simulink model "mloc_estimation_postprocessing"  (R2018b)
settings: configuration reference "Active" (kept outside this file)
model workspace (MAT data in the model file):
  P_VDC_LocalizationMode = Simulink.Parameter
  P_VDC_LocalizationMode.Value = 1
  P_VDC_LocalizationMode.DataType = 'auto'
  P_VDC_LocalizationMode.Dimensions = [1 1]
undefined symbols (not defined in the file): l_front_m, l_rear_m, P_MLOC_MaxWheelslip_perc, P_MLOC_MaxWheelslipangle_rad, P_MLOC_MinWheelslip_perc, P_MLOC_MinWheelslipangle_rad, P_MLOC_OdometryMode, P_MLOC_OdometrySwitchSpeed_mps, P_MLOC_VLOCManualReset_psi_rad, P_MLOC_VLOCManualReset_x_m, P_MLOC_VLOCManualReset_y_m, P_MLOC_VLOCResetMode, P_VDC_CurvatureEstimateMax_radpm, P_VDC_CurvatureEstimationMode, P_VDC_LowPassT1Curvature, P_VDC_MinVelSlipCalc_mps, P_VDC_resLim_dGPS_m, P_VDC_resLim_dVLOC_m, P_VDC_resLim_psiGPS_rad, P_VDC_resLim_psiVLOC_rad, P_VDC_resLim_sGPS_m, P_VDC_resLim_sVLOC_m, P_VDC_resLim_vx_mps, P_VDC_resLim_vy_mps, tS, TUMOdometryEstimationState, TUMStateEstimationState, tw_front_m, tw_rear_m, tyreradius_front_m, tyreradius_rear_m
libraries: simulink x11, rr_general x4
settings Model: DataDictionary=mloc_estimation_postprocessing.sldd  ParameterArgumentNames=P_VDC_LocalizationMode  Creator=wischnewski  LastModifiedBy=ge34qer

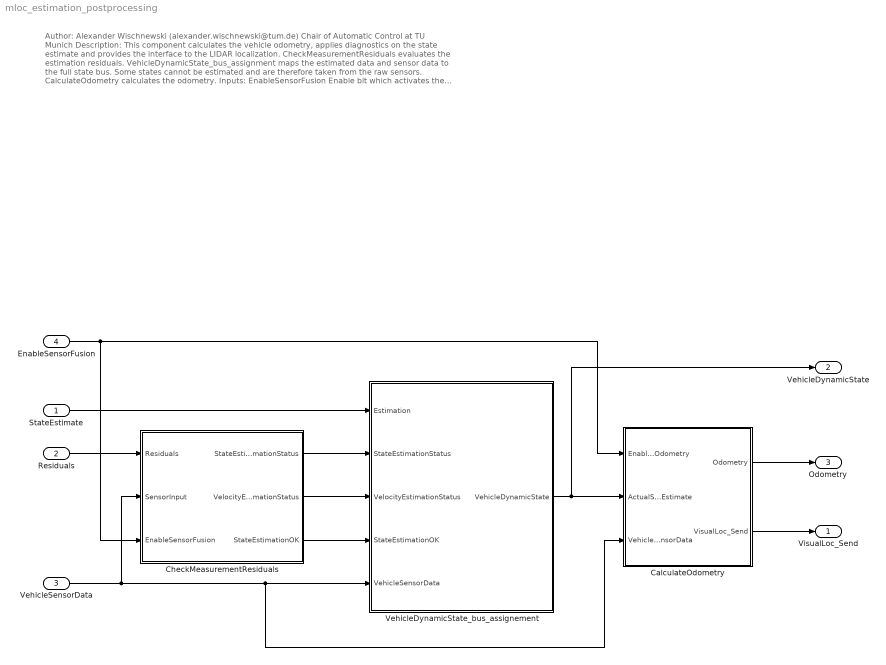
== system mloc_estimation_postprocessing ==
  note: Author: Alexander Wischnewski (alexander.wischnewski@tum.de)
      | Chair of Automatic Control at TU Munich
      |
      | Description: This component calculates the vehicle odometry, applies diagnostics on the state estimate and provides the interface to the LIDAR localization.
      |
      | CheckMeasurementResiduals evaluates the estimation residuals.
      |
      | VehicleDynamicState_bus_assignment maps the estimated data and sensor data to the full state bus. Some states cannot be estimated and are therefore taken from the raw sensors.
      |
      | CalculateOdometry calculates the odometry.
      |
      | Inputs:
      | EnableSensorFusion Enable bit which activates the Kalman Filter
      | StateEstimate State estimation vector from the Kalman Filter
      | Residuals Residual vector of the Kalman Filter
      | VehicleSensorData raw sensor data
      |
      | Outputs:
      | VehicleDynamicState Estimate of the vehicle dynamic state (best available)
      | VisualLocSend Data which is send to the LIDAR localization algorithm
      | Odometry Vehicle odometry as forward integrated position
  "StateEstimate " : Inport  OutDataTypeStr=Bus: StateEstimation_state  BusOutputAsStruct=on
  Residuals : Inport  Port=2  OutDataTypeStr=Bus: StateEstimation_residuals  BusOutputAsStruct=on
  VehicleSensorData : Inport  Port=3  OutDataTypeStr=Bus: VehicleSensorData  BusOutputAsStruct=on
  EnableSensorFusion : Inport  Port=4  OutDataTypeStr=boolean  BusOutputAsStruct=on
  CalculateOdometry : Subsystem
  CheckMeasurementResiduals : Subsystem
  VehicleDynamicState_bus_assignement : Subsystem
  VisualLoc_Send : Outport  OutDataTypeStr=Bus: VisualLoc_Send  BusOutputAsStruct=on
  VehicleDynamicState : Outport  Port=2  OutDataTypeStr=Bus: VehicleDynamicState  BusOutputAsStruct=on
  Odometry : Outport  Port=3  OutDataTypeStr=Bus: Odometry  BusOutputAsStruct=on
  wires:
  VehicleDynamicState_bus_assignement/1(VehicleDynamicState) -> VehicleDynamicState/1, CalculateOdometry/2(ActualStateEstimate)
  CalculateOdometry/2(VisualLoc_Send) -> VisualLoc_Send/1
  EnableSensorFusion/1 -> CalculateOdometry/1(EnableOdometry), CheckMeasurementResiduals/3(EnableSensorFusion)
  CheckMeasurementResiduals/1(StateEstimationStatus) -> VehicleDynamicState_bus_assignement/2(StateEstimationStatus)
  CheckMeasurementResiduals/2(VelocityEstimationStatus) -> VehicleDynamicState_bus_assignement/3(VelocityEstimationStatus)
  CheckMeasurementResiduals/3(StateEstimationOK) -> VehicleDynamicState_bus_assignement/4(StateEstimationOK)
  "StateEstimate "/1 -> VehicleDynamicState_bus_assignement/1(Estimation)
  CalculateOdometry/1(Odometry) -> Odometry/1
  VehicleSensorData/1 -> CheckMeasurementResiduals/2(SensorInput), CalculateOdometry/3(VehicleSensorData), VehicleDynamicState_bus_assignement/5(VehicleSensorData)
  Residuals/1 -> CheckMeasurementResiduals/1(Residuals)

== system mloc_estimation_postprocessing/CalculateOdometry ==
  note: calculates an Odometry based on
      | the vehicle motion sensors. Different options are available.
      | Check "Integrate Odometry" for details.
  EnableOdometry : Inport
  ActualStateEstimate : Inport  Port=2
  VehicleSensorData : Inport  Port=3
  DetermineResetPosition : Subsystem
  IntegrateOdometry : Subsystem
  VisualLocalizationInterface : Subsystem
  Odometry : Outport
  VisualLoc_Send : Outport  Port=2  OutDataTypeStr=Bus: VisualLoc_Send  BusOutputAsStruct=on
  wires:
  IntegrateOdometry/1(Odometry) -> VisualLocalizationInterface/1(Odometry), Odometry/1
  DetermineResetPosition/2(ResetPositionValid_b) -> VisualLocalizationInterface/3(ResetPosition_Valid), IntegrateOdometry/4(ResetPositionValid)
  DetermineResetPosition/1(ResetPosition) -> VisualLocalizationInterface/2(ResetPosition), IntegrateOdometry/3(ResetPosition)
  VehicleSensorData/1 -> VisualLocalizationInterface/5(VehicleSensorData), IntegrateOdometry/5(VehicleSensors), DetermineResetPosition/2(VehicleSensorData)
  EnableOdometry/1 -> IntegrateOdometry/1(EnableOdometry)
  ActualStateEstimate/1 -> VisualLocalizationInterface/4(VehicleDynamicState), IntegrateOdometry/2(ActualStateEstimate), DetermineResetPosition/1(StateEstimate)
  VisualLocalizationInterface/1(VisualLoc_Send) -> VisualLoc_Send/1

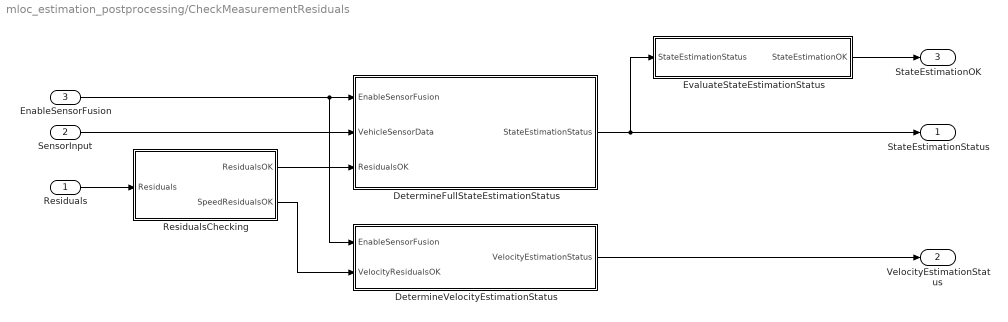
== system mloc_estimation_postprocessing/CheckMeasurementResiduals ==
  Residuals : Inport
  SensorInput : Inport  Port=2
  EnableSensorFusion : Inport  Port=3
  DetermineFullStateEstimationStatus : Subsystem
  DetermineVelocityEstimationStatus : Subsystem
  EvaluateStateEstimationStatus : Subsystem
  ResidualsChecking : Subsystem
  StateEstimationStatus : Outport
  VelocityEstimationStatus : Outport  Port=2
  StateEstimationOK : Outport  Port=3
  wires:
  Residuals/1 -> ResidualsChecking/1(Residuals)
  EnableSensorFusion/1 -> DetermineVelocityEstimationStatus/1(EnableSensorFusion), DetermineFullStateEstimationStatus/1(EnableSensorFusion)
  EvaluateStateEstimationStatus/1(StateEstimationOK) -> StateEstimationOK/1
  ResidualsChecking/2(SpeedResidualsOK) -> DetermineVelocityEstimationStatus/2(VelocityResidualsOK)
  DetermineVelocityEstimationStatus/1(VelocityEstimationStatus) -> VelocityEstimationStatus/1
  DetermineFullStateEstimationStatus/1(StateEstimationStatus) -> StateEstimationStatus/1, EvaluateStateEstimationStatus/1(StateEstimationStatus)
  SensorInput/1 -> DetermineFullStateEstimationStatus/2(VehicleSensorData)
  ResidualsChecking/1(ResidualsOK) -> DetermineFullStateEstimationStatus/3(ResidualsOK)

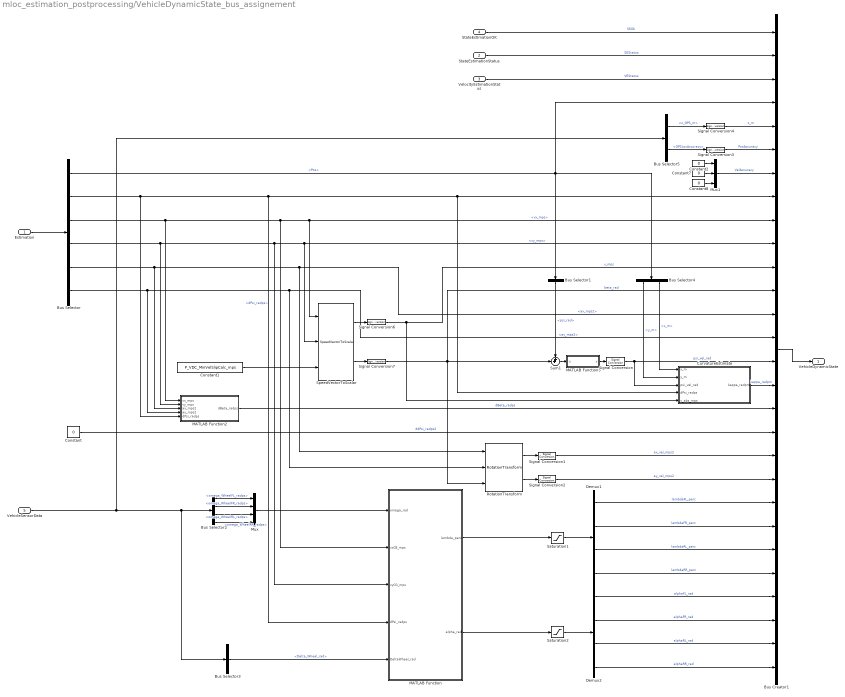
== system mloc_estimation_postprocessing/VehicleDynamicState_bus_assignement ==
  Estimation : Inport
  StateEstimationStatus : Inport  Port=2
  VelocityEstimationStatus : Inport  Port=3
  StateEstimationOK : Inport  Port=4
  VehicleSensorData : Inport  Port=5
  Bus Creator1 : BusCreator  Inputs=28
  Bus Selector : BusSelector  OutputSignals=Pos,dPsi_radps,vx_mps,vy_mps,ax_mps2,ay_mps2
  Bus Selector1 : BusSelector  OutputSignals=psi_rad
  Bus Selector2 : BusSelector  OutputSignals=omega_WheelFL_radps,omega_WheelFR_radps,omega_WheelRL_radps,omega_WheelRR_radps
  Bus Selector3 : BusSelector  OutputSignals=Delta_Wheel_rad
  Bus Selector4 : BusSelector  OutputSignals=y_m,x_m
  Bus Selector5 : BusSelector  OutputSignals=z_GPS_m,GPSLocAccuracy
  Constant{,2,7..8} (4 alike) : Constant  Value=0
  Constant1 : Constant  Value=P_VDC_MinVelSlipCalc_mps
  CurvatureEstimate : Subsystem
  Demux1 : Demux
  Demux2 : Demux
  MATLAB Function : MATLAB Function  TreatAsAtomicUnit=on
  MATLAB Function2 : MATLAB Function  TreatAsAtomicUnit=on
  MATLAB Function3 : MATLAB Function  TreatAsAtomicUnit=on
  Mux : Mux
  Mux1 : Mux  Inputs=3
  RotationTransform : rr_general/RotationTransform  SystemSampleTime=-1
  Saturation1 : Saturate  UpperLimit=P_MLOC_MaxWheelslip_perc  LowerLimit=P_MLOC_MinWheelslip_perc
  Saturation2 : Saturate  UpperLimit=P_MLOC_MaxWheelslipangle_rad  LowerLimit=P_MLOC_MinWheelslipangle_rad
  Signal Conversion{,1..4,6..7} (7 alike) : SignalConversion  OverrideOpt=off
  SpeedVectorToScalar : rr_general/SpeedVectorToScalar  SystemSampleTime=-1
  Sum1 : Sum  Inputs=++|
  VehicleDynamicState : Outport
  wires:
  Bus Creator1/1 -> VehicleDynamicState/1
  Sum1/1 -> MATLAB Function3/1(u)
  Bus Selector/3 -> MATLAB Function2/1(vx_mps), MATLAB Function/2(vxCB_mps), SpeedVectorToScalar/1, Bus Creator1/9  "<vx_mps>"
  Bus Selector/1 -> Bus Selector4/1, Bus Creator1/4, Bus Selector1/1  "<Pos>"
  Bus Selector1/1 -> Sum1/1  "<psi_rad>"
  Estimation/1 -> Bus Selector/1
  StateEstimationStatus/1 -> Bus Creator1/2  "SEStatus"
  MATLAB Function3/1(y) -> Signal Conversion/1
  CurvatureEstimate/1(kappa_radpm) -> Bus Creator1/16  "kappa_radpm"
  Signal Conversion/1 -> Bus Creator1/15, CurvatureEstimate/3(psi_vel_rad)  "psi_vel_rad"
  MATLAB Function2/1(dBeta_radps) -> Bus Creator1/17  "dBeta_radps"
  Constant/1 -> Bus Creator1/18  "ddPsi_radps2"
  Bus Selector/4 -> MATLAB Function/3(vyCG_mps), Bus Creator1/10, SpeedVectorToScalar/2, MATLAB Function2/2(vy_mps)  "<vy_mps>"
  SpeedVectorToScalar/1 -> Signal Conversion6/1
  SpeedVectorToScalar/2 -> Signal Conversion7/1
  Signal Conversion6/1 -> Bus Creator1/11, CurvatureEstimate/5(v_abs_mps)  "v_mps"
  Bus Selector/5 -> MATLAB Function2/3(ax_mps2), RotationTransform/1, Bus Creator1/13  "<ax_mps2>"
  Bus Selector/6 -> RotationTransform/2, Bus Creator1/14, MATLAB Function2/4(ay_mps2)  "<ay_mps2>"
  Signal Conversion7/1 -> Sum1/2, RotationTransform/3, Bus Creator1/12  "beta_rad"
  RotationTransform/1 -> Signal Conversion1/1
  RotationTransform/2 -> Signal Conversion2/1
  Signal Conversion1/1 -> Bus Creator1/19  "ax_vel_mps2"
  Signal Conversion2/1 -> Bus Creator1/20  "ay_vel_mps2"
  VelocityEstimationStatus/1 -> Bus Creator1/3  "VEStatus"
  Bus Selector/2 -> MATLAB Function2/5(dPsi_radps), MATLAB Function/4(dPsi_radps), Bus Creator1/8, CurvatureEstimate/4(dPsi_radps)  "<dPsi_radps>"
  MATLAB Function/1(lambda_perc) -> Saturation1/1
  MATLAB Function/2(alpha_rad) -> Saturation2/1
  Saturation1/1 -> Demux1/1
  Saturation2/1 -> Demux2/1
  Demux2/1 -> Bus Creator1/25  "alphaFL_rad"
  Demux2/2 -> Bus Creator1/26  "alphaFR_rad"
  Demux2/3 -> Bus Creator1/27  "alphaRL_rad"
  Demux2/4 -> Bus Creator1/28  "alphaRR_rad"
  Demux1/1 -> Bus Creator1/21  "lambdaFL_perc"
  Demux1/2 -> Bus Creator1/22  "lambdaFR_perc"
  Demux1/3 -> Bus Creator1/23  "lambdaRL_perc"
  Demux1/4 -> Bus Creator1/24  "lambdaRR_perc"
  VehicleSensorData/1 -> Bus Selector5/1, Bus Selector3/1, Bus Selector2/1
  Bus Selector2/1 -> Mux/1  "<omega_WheelFL_radps>"
  Bus Selector2/2 -> Mux/2  "<omega_WheelFR_radps>"
  Bus Selector2/3 -> Mux/3  "<omega_WheelRL_radps>"
  Bus Selector2/4 -> Mux/4  "<omega_WheelRR_radps>"
  Mux/1 -> MATLAB Function/1(omega_rad)
  Bus Selector3/1 -> MATLAB Function/5(DeltaWheel_rad)  "<Delta_Wheel_rad>"
  StateEstimationOK/1 -> Bus Creator1/1  "SEOk"
  Constant1/1 -> SpeedVectorToScalar/3
  Bus Selector4/1 -> CurvatureEstimate/2(y_m)  "<y_m>"
  Bus Selector4/2 -> CurvatureEstimate/1("x_m ")  "<x_m>"
  Bus Selector5/2 -> Signal Conversion3/1  "<GPSLocAccuracy>"
  Constant8/1 -> Mux1/3
  Mux1/1 -> Bus Creator1/7  "VelAccuracy"
  Constant2/1 -> Mux1/1
  Constant7/1 -> Mux1/2
  Signal Conversion3/1 -> Bus Creator1/6  "PosAccuracy"
  Bus Selector5/1 -> Signal Conversion4/1  "<z_GPS_m>"
  Signal Conversion4/1 -> Bus Creator1/5  "z_m"

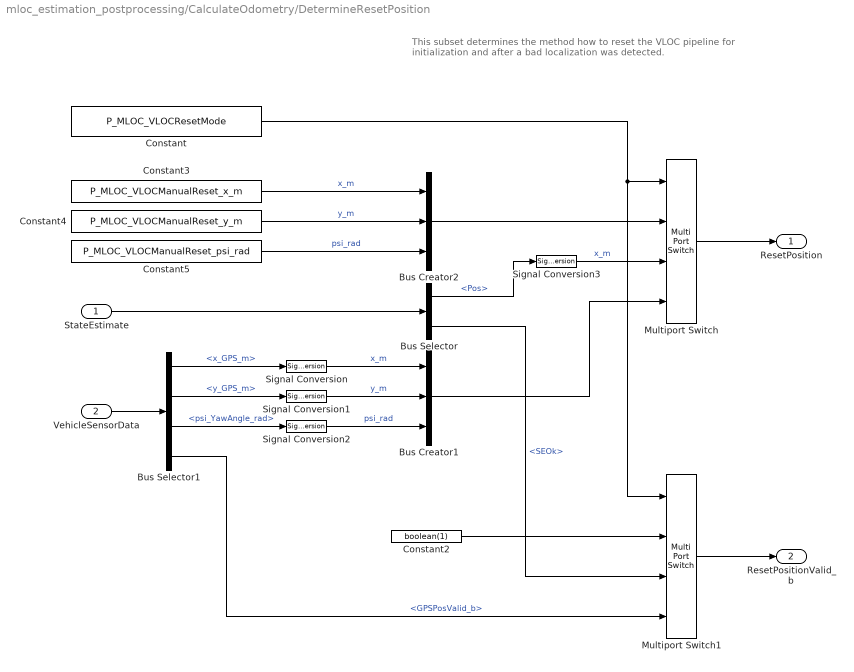
== system mloc_estimation_postprocessing/CalculateOdometry/DetermineResetPosition ==
  note: This subset determines the method how to reset the
      | VLOC pipeline for initialization and after a bad localization was detected.
  StateEstimate : Inport
  VehicleSensorData : Inport  Port=2
  Bus Creator1 : BusCreator  Inputs=3  OutDataTypeStr=Bus: CartPos
  Bus Creator2 : BusCreator  Inputs=3  OutDataTypeStr=Bus: CartPos
  Bus Selector : BusSelector  OutputSignals=Pos,SEOk
  Bus Selector1 : BusSelector  OutputSignals=x_GPS_m,y_GPS_m,psi_YawAngle_rad,GPSPosValid_b
  Constant : Constant  Value=P_MLOC_VLOCResetMode
  Constant2 : Constant  Value=boolean(1)
  Constant3 : Constant  Value=P_MLOC_VLOCManualReset_x_m
  Constant4 : Constant  Value=P_MLOC_VLOCManualReset_y_m
  Constant5 : Constant  Value=P_MLOC_VLOCManualReset_psi_rad
  Multiport Switch : MultiPortSwitch
  Multiport Switch1 : MultiPortSwitch
  Signal Conversion : SignalConversion  OverrideOpt=off
  Signal Conversion1 : SignalConversion  OverrideOpt=off
  Signal Conversion2 : SignalConversion  OverrideOpt=off
  Signal Conversion3 : SignalConversion  ConversionOutput=Virtual bus  OverrideOpt=off
  ResetPosition : Outport
  ResetPositionValid_b : Outport  Port=2
  wires:
  Constant3/1 -> Bus Creator2/1  "x_m"
  Constant4/1 -> Bus Creator2/2  "y_m"
  Constant5/1 -> Bus Creator2/3  "psi_rad"
  Bus Creator2/1 -> Multiport Switch/2
  StateEstimate/1 -> Bus Selector/1
  Bus Selector/1 -> Signal Conversion3/1  "<Pos>"
  VehicleSensorData/1 -> Bus Selector1/1
  Signal Conversion/1 -> Bus Creator1/1  "x_m"
  Bus Selector1/1 -> Signal Conversion/1  "<x_GPS_m>"
  Bus Selector1/2 -> Signal Conversion1/1  "<y_GPS_m>"
  Bus Selector1/3 -> Signal Conversion2/1  "<psi_YawAngle_rad>"
  Signal Conversion2/1 -> Bus Creator1/3  "psi_rad"
  Signal Conversion1/1 -> Bus Creator1/2  "y_m"
  Bus Creator1/1 -> Multiport Switch/4
  Multiport Switch/1 -> ResetPosition/1
  Multiport Switch1/1 -> ResetPositionValid_b/1
  Constant2/1 -> Multiport Switch1/2
  Bus Selector1/4 -> Multiport Switch1/4  "<GPSPosValid_b>"
  Bus Selector/2 -> Multiport Switch1/3  "<SEOk>"
  Constant/1 -> Multiport Switch/1, Multiport Switch1/1
  Signal Conversion3/1 -> Multiport Switch/3  "x_m"

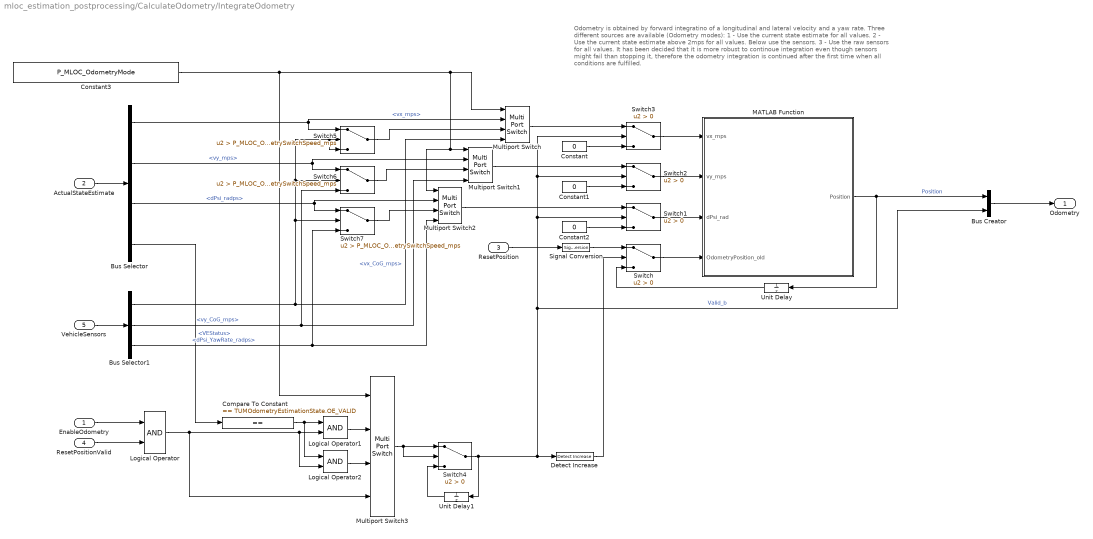
== system mloc_estimation_postprocessing/CalculateOdometry/IntegrateOdometry ==
  note: Odometry is obtained by forward integratino of a longitudinal and lateral velocity and a yaw rate.
      | Three different sources are available (Odometry modes):
      | 1 - Use the current state estimate for all values.
      | 2 - Use the current state estimate above 2mps for all values. Below use the sensors.
      | 3 - Use the raw sensors for all values.
      |
      | It has been decided that it is more robust to continoue integration even though sensors might fail than stopping it,
      | therefore the odometry integration is continued after the first time when all conditions are fulfilled.
  EnableOdometry : Inport
  ActualStateEstimate : Inport  Port=2
  ResetPosition : Inport  Port=3
  ResetPositionValid : Inport  Port=4
  VehicleSensors : Inport  Port=5
  Bus Creator : BusCreator  Inputs=2
  Bus Selector : BusSelector  OutputSignals=vx_mps,vy_mps,dPsi_radps,VEStatus
  Bus Selector1 : BusSelector  OutputSignals=vx_CoG_mps,vy_CoG_mps,dPsi_YawRate_radps
  Compare To Constant : simulink/Logic and Bit Operations/Compare To Constant  relop===  const=TUMOdometryEstimationState.OE_VALID  OutDataTypeStr=boolean
  Constant : Constant  Value=0
  Constant1 : Constant  Value=0
  Constant2 : Constant  Value=0
  Constant3 : Constant  Value=P_MLOC_OdometryMode
  Detect Increase : simulink/Logic and Bit Operations/Detect Increase  vinit=0.0  OutDataTypeStr=boolean
  Logical Operator : Logic  AllPortsSameDT=off  OutDataTypeStr=boolean
  Logical Operator1 : Logic  AllPortsSameDT=off  OutDataTypeStr=boolean
  Logical Operator2 : Logic  AllPortsSameDT=off  OutDataTypeStr=boolean
  MATLAB Function : MATLAB Function  TreatAsAtomicUnit=on
  Multiport Switch{,1..3} (4 alike) : MultiPortSwitch
  Signal Conversion : SignalConversion  ConversionOutput=Nonvirtual bus  OverrideOpt=off
  Switch{,1..4} (5 alike) : Switch  Criteria=u2 > Threshold
  Switch5 : Switch  Criteria=u2 > Threshold  Threshold=P_MLOC_OdometrySwitchSpeed_mps
  Switch6 : Switch  Criteria=u2 > Threshold  Threshold=P_MLOC_OdometrySwitchSpeed_mps
  Switch7 : Switch  Criteria=u2 > Threshold  Threshold=P_MLOC_OdometrySwitchSpeed_mps
  Unit Delay : UnitDelay  SampleTime=-1
  Unit Delay1 : UnitDelay  SampleTime=-1
  Odometry : Outport  BusOutputAsStruct=on
  wires:
  ActualStateEstimate/1 -> Bus Selector/1
  Switch/1 -> MATLAB Function/4(OdometryPosition_old)
  Unit Delay/1 -> Switch/3
  Switch1/1 -> MATLAB Function/3(dPsi_rad)
  Switch2/1 -> MATLAB Function/2(vy_mps)
  Switch3/1 -> MATLAB Function/1(vx_mps)
  Constant/1 -> Switch3/3
  Constant1/1 -> Switch2/3
  Constant2/1 -> Switch1/3
  Multiport Switch3/1 -> Switch4/2, Switch4/1
  Unit Delay1/1 -> Switch4/3
  Switch4/1 -> Detect Increase/1, Bus Creator/2, Switch3/2, Switch2/2, Switch1/2, Unit Delay1/1  "Valid_b"
  Detect Increase/1 -> Switch/2
  MATLAB Function/1(Position) -> Unit Delay/1, Bus Creator/1  "Position"
  Bus Creator/1 -> Odometry/1
  Multiport Switch/1 -> Switch3/1
  Multiport Switch1/1 -> Switch2/1
  Multiport Switch2/1 -> Switch1/1
  VehicleSensors/1 -> Bus Selector1/1
  Bus Selector/1 -> Multiport Switch/2, Switch5/1  "<vx_mps>"
  Bus Selector/2 -> Multiport Switch1/2, Switch6/1  "<vy_mps>"
  Bus Selector/3 -> Multiport Switch2/2, Switch7/1  "<dPsi_radps>"
  Bus Selector1/3 -> Switch7/3, Multiport Switch2/4  "<dPsi_YawRate_radps>"
  Bus Selector1/2 -> Switch6/3, Multiport Switch1/4  "<vy_CoG_mps>"
  Bus Selector1/1 -> Switch7/2, Switch6/2, Switch5/3, Switch5/2, Multiport Switch/4  "<vx_CoG_mps>"
  Switch5/1 -> Multiport Switch/3
  Switch6/1 -> Multiport Switch1/3
  Switch7/1 -> Multiport Switch2/3
  Constant3/1 -> Multiport Switch3/1, Multiport Switch1/1, Multiport Switch2/1, Multiport Switch/1
  EnableOdometry/1 -> Logical Operator/1
  ResetPositionValid/1 -> Logical Operator/2
  Logical Operator1/1 -> Multiport Switch3/2
  Logical Operator/1 -> Multiport Switch3/4, Logical Operator2/2, Logical Operator1/2
  Compare To Constant/1 -> Logical Operator2/1, Logical Operator1/1
  Bus Selector/4 -> Compare To Constant/1  "<VEStatus>"
  Logical Operator2/1 -> Multiport Switch3/3
  Signal Conversion/1 -> Switch/1
  ResetPosition/1 -> Signal Conversion/1

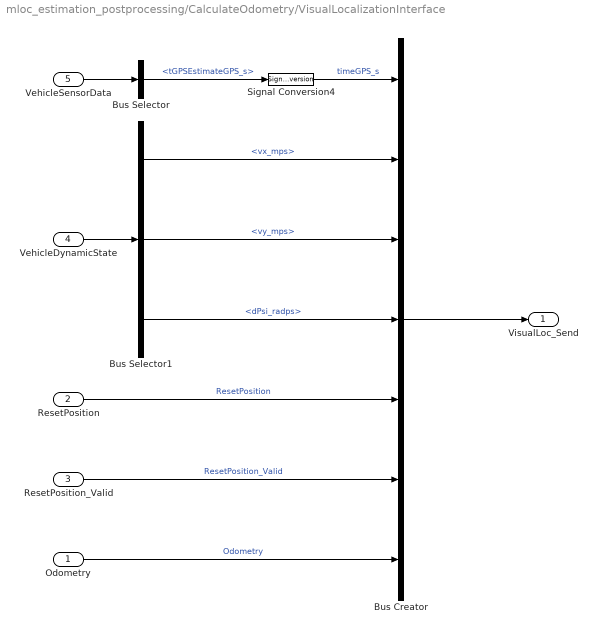
== system mloc_estimation_postprocessing/CalculateOdometry/VisualLocalizationInterface ==
  Odometry : Inport
  ResetPosition : Inport  Port=2
  ResetPosition_Valid : Inport  Port=3
  VehicleDynamicState : Inport  Port=4
  VehicleSensorData : Inport  Port=5
  Bus Creator : BusCreator  Inputs=7
  Bus Selector : BusSelector  OutputSignals=tGPSEstimateGPS_s
  Bus Selector1 : BusSelector  OutputSignals=vx_mps,vy_mps,dPsi_radps
  Signal Conversion4 : SignalConversion  OverrideOpt=off
  VisualLoc_Send : Outport  BusOutputAsStruct=on
  wires:
  Bus Creator/1 -> VisualLoc_Send/1
  VehicleSensorData/1 -> Bus Selector/1
  Bus Selector/1 -> Signal Conversion4/1  "<tGPSEstimateGPS_s>"
  Signal Conversion4/1 -> Bus Creator/1  "timeGPS_s"
  VehicleDynamicState/1 -> Bus Selector1/1
  Bus Selector1/1 -> Bus Creator/2  "<vx_mps>"
  Bus Selector1/2 -> Bus Creator/3  "<vy_mps>"
  Bus Selector1/3 -> Bus Creator/4  "<dPsi_radps>"
  ResetPosition/1 -> Bus Creator/5  "ResetPosition"
  ResetPosition_Valid/1 -> Bus Creator/6  "ResetPosition_Valid"
  Odometry/1 -> Bus Creator/7  "Odometry"

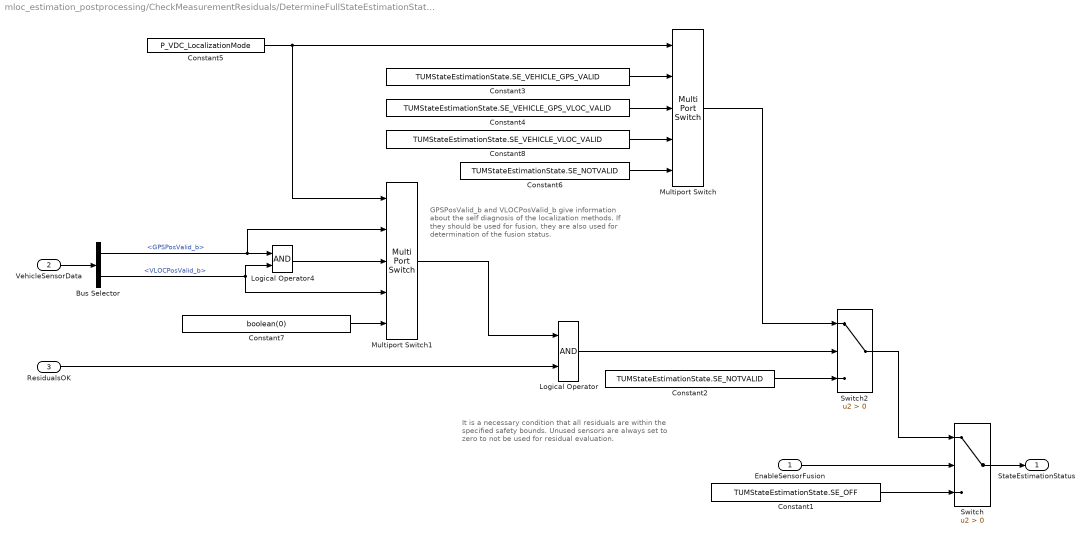
== system mloc_estimation_postprocessing/CheckMeasurementResiduals/DetermineFullStateEstimationStatus ==
  note: It is a necessary condition that all residuals are within
      | the specified safety bounds. Unused sensors are always
      | set to zero to not be used for residual evaluation.
  note: GPSPosValid_b and VLOCPosValid_b
      | give information about the self diagnosis of the
      | localization methods.
      | If they should be used for fusion, they are also used
      | for determination of the fusion status.
  EnableSensorFusion : Inport
  VehicleSensorData : Inport  Port=2
  ResidualsOK : Inport  Port=3
  Bus Selector : BusSelector  OutputSignals=GPSPosValid_b,VLOCPosValid_b
  Constant1 : Constant  Value=TUMStateEstimationState.SE_OFF
  Constant2 : Constant  Value=TUMStateEstimationState.SE_NOTVALID
  Constant3 : Constant  Value=TUMStateEstimationState.SE_VEHICLE_GPS_VALID
  Constant4 : Constant  Value=TUMStateEstimationState.SE_VEHICLE_GPS_VLOC_VALID
  Constant5 : Constant  Value=P_VDC_LocalizationMode
  Constant6 : Constant  Value=TUMStateEstimationState.SE_NOTVALID
  Constant7 : Constant  Value=boolean(0)
  Constant8 : Constant  Value=TUMStateEstimationState.SE_VEHICLE_VLOC_VALID
  Logical Operator : Logic  AllPortsSameDT=off  OutDataTypeStr=boolean
  Logical Operator4 : Logic  AllPortsSameDT=off  OutDataTypeStr=boolean
  Multiport Switch : MultiPortSwitch  DataPortOrder=Zero-based contiguous  Inputs=4  zeroidx=on
  Multiport Switch1 : MultiPortSwitch  DataPortOrder=Zero-based contiguous  Inputs=4  zeroidx=on
  Switch : Switch  Criteria=u2 > Threshold
  Switch2 : Switch  Criteria=u2 > Threshold
  StateEstimationStatus : Outport
  wires:
  EnableSensorFusion/1 -> Switch/2
  Constant2/1 -> Switch2/3
  Logical Operator/1 -> Switch2/2
  Switch2/1 -> Switch/1
  Switch/1 -> StateEstimationStatus/1
  Constant1/1 -> Switch/3
  ResidualsOK/1 -> Logical Operator/2
  Multiport Switch/1 -> Switch2/1
  VehicleSensorData/1 -> Bus Selector/1
  Constant3/1 -> Multiport Switch/2
  Constant8/1 -> Multiport Switch/4
  Constant4/1 -> Multiport Switch/3
  Constant5/1 -> Multiport Switch1/1, Multiport Switch/1
  Constant6/1 -> Multiport Switch/5
  Multiport Switch1/1 -> Logical Operator/1
  Bus Selector/1 -> Multiport Switch1/2, Logical Operator4/1  "<GPSPosValid_b>"
  Bus Selector/2 -> Multiport Switch1/4, Logical Operator4/2  "<VLOCPosValid_b>"
  Logical Operator4/1 -> Multiport Switch1/3
  Constant7/1 -> Multiport Switch1/5

== system mloc_estimation_postprocessing/CheckMeasurementResiduals/DetermineVelocityEstimationStatus ==
  note: determines if the velocity states of the sensor fusion are ok.
      | This is necessary as the odometry must start before the LIDAR localization
      | is ready. The full state estimation therefore requires
      | a valid odometry to power up in case LIDAR is used.
  EnableSensorFusion : Inport
  VelocityResidualsOK : Inport  Port=2
  Constant5 : Constant  Value=TUMOdometryEstimationState.OE_OFF
  Constant6 : Constant  Value=TUMOdometryEstimationState.OE_NOTVALID
  Constant7 : Constant  Value=TUMOdometryEstimationState.OE_VALID
  Switch3 : Switch  Criteria=u2 > Threshold
  Switch4 : Switch  Criteria=u2 > Threshold
  VelocityEstimationStatus : Outport
  wires:
  EnableSensorFusion/1 -> Switch3/2
  Constant5/1 -> Switch3/3
  Switch4/1 -> Switch3/1
  VelocityResidualsOK/1 -> Switch4/2
  Constant6/1 -> Switch4/3
  Constant7/1 -> Switch4/1
  Switch3/1 -> VelocityEstimationStatus/1

== system mloc_estimation_postprocessing/CheckMeasurementResiduals/EvaluateStateEstimationStatus ==
  note: evaluates the self diagnosis of
      | the sensor fusion and outputs
      | an OK or not OK bit dependent
      | on the required localization mode.
  StateEstimationStatus : Inport
  Compare To Constant : simulink/Logic and Bit Operations/Compare To Constant  relop===  const=TUMStateEstimationState.SE_VEHICLE_GPS_VALID  OutDataTypeStr=boolean
  Compare To Constant1 : simulink/Logic and Bit Operations/Compare To Constant  relop===  const=TUMStateEstimationState.SE_VEHICLE_VLOC_VALID  OutDataTypeStr=boolean
  Compare To Constant2 : simulink/Logic and Bit Operations/Compare To Constant  relop===  const=TUMStateEstimationState.SE_VEHICLE_GPS_VLOC_VALID  OutDataTypeStr=boolean
  Constant9 : Constant  Value=P_VDC_LocalizationMode
  Logical Operator2 : Logic  Operator=OR  Inputs=3  AllPortsSameDT=off  OutDataTypeStr=boolean
  Multiport Switch : MultiPortSwitch  DataPortOrder=Zero-based contiguous  zeroidx=on
  StateEstimationOK : Outport
  wires:
  StateEstimationStatus/1 -> Compare To Constant1/1, Compare To Constant2/1, Compare To Constant/1
  Multiport Switch/1 -> StateEstimationOK/1
  Constant9/1 -> Multiport Switch/1
  Compare To Constant/1 -> Multiport Switch/2, Logical Operator2/1
  Logical Operator2/1 -> Multiport Switch/3
  Compare To Constant1/1 -> Logical Operator2/2, Multiport Switch/4
  Compare To Constant2/1 -> Logical Operator2/3

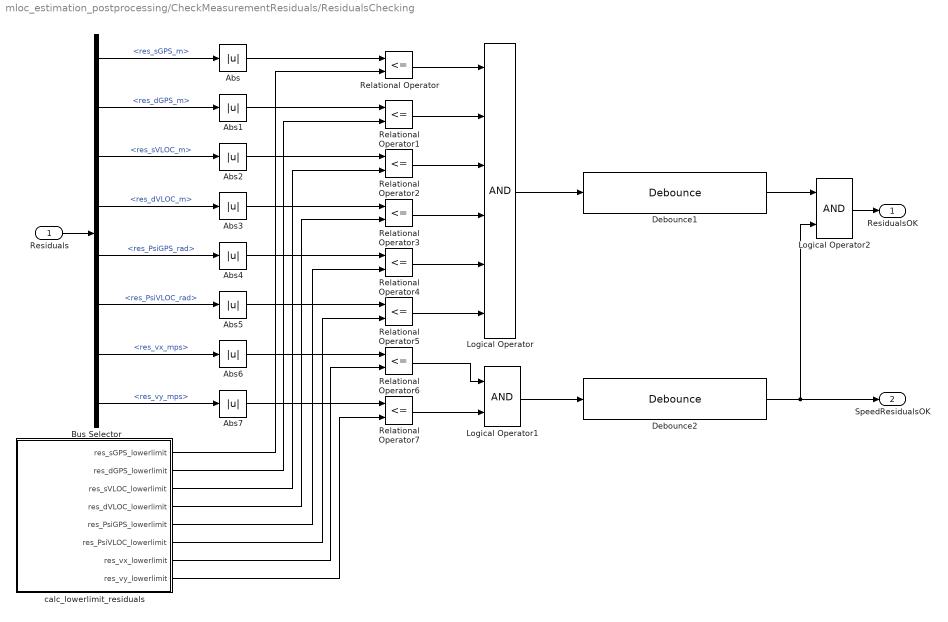
== system mloc_estimation_postprocessing/CheckMeasurementResiduals/ResidualsChecking ==
  Residuals : Inport
  Abs{,1..7} (8 alike) : Abs
  Bus Selector : BusSelector  OutputSignals=res_sGPS_m,res_dGPS_m,res_sVLOC_m,res_dVLOC_m,res_PsiGPS_rad,res_PsiVLOC_rad,res_vx_mps,res_vy_mps
  Debounce1 : rr_general/Debounce  debounce_cycles=P_VDC_ResidualsDebounceCounterPositionMax
  Debounce2 : rr_general/Debounce  debounce_cycles=P_VDC_ResidualsDebounceCounterVelocityMax
  Logical Operator : Logic  Inputs=6  AllPortsSameDT=off  OutDataTypeStr=boolean
  Logical Operator1 : Logic  AllPortsSameDT=off  OutDataTypeStr=boolean
  Logical Operator2 : Logic  AllPortsSameDT=off  OutDataTypeStr=boolean
  Relational Operator{,1..7} (8 alike) : RelationalOperator  Operator=<=  OutDataTypeStr=boolean  RndMeth=Nearest
  calc_lowerlimit_residuals : Subsystem
  ResidualsOK : Outport
  SpeedResidualsOK : Outport  Port=2
  wires:
  Relational Operator4/1 -> Logical Operator/5
  Bus Selector/2 -> Abs1/1  "<res_dGPS_m>"
  Bus Selector/4 -> Abs3/1  "<res_dVLOC_m>"
  Bus Selector/5 -> Abs4/1  "<res_PsiGPS_rad>"
  Relational Operator3/1 -> Logical Operator/4
  Relational Operator2/1 -> Logical Operator/3
  Relational Operator1/1 -> Logical Operator/2
  Bus Selector/6 -> Abs5/1  "<res_PsiVLOC_rad>"
  Bus Selector/7 -> Abs6/1  "<res_vx_mps>"
  Bus Selector/3 -> Abs2/1  "<res_sVLOC_m>"
  Relational Operator/1 -> Logical Operator/1
  Residuals/1 -> Bus Selector/1
  Bus Selector/1 -> Abs/1  "<res_sGPS_m>"
  Relational Operator6/1 -> Logical Operator1/1
  Relational Operator5/1 -> Logical Operator/6
  Relational Operator7/1 -> Logical Operator1/2
  Bus Selector/8 -> Abs7/1  "<res_vy_mps>"
  Abs/1 -> Relational Operator/1
  Abs6/1 -> Relational Operator6/1
  Abs7/1 -> Relational Operator7/1
  Abs4/1 -> Relational Operator4/1
  Abs2/1 -> Relational Operator2/1
  Abs1/1 -> Relational Operator1/1
  Abs5/1 -> Relational Operator5/1
  Abs3/1 -> Relational Operator3/1
  calc_lowerlimit_residuals/1(res_sGPS_lowerlimit) -> Relational Operator/2
  calc_lowerlimit_residuals/2(res_dGPS_lowerlimit) -> Relational Operator1/2
  calc_lowerlimit_residuals/3(res_sVLOC_lowerlimit) -> Relational Operator2/2
  calc_lowerlimit_residuals/4(res_dVLOC_lowerlimit) -> Relational Operator3/2
  calc_lowerlimit_residuals/5(res_PsiGPS_lowerlimit) -> Relational Operator4/2
  calc_lowerlimit_residuals/6(res_PsiVLOC_lowerlimit) -> Relational Operator5/2
  calc_lowerlimit_residuals/7(res_vx_lowerlimit) -> Relational Operator6/2
  calc_lowerlimit_residuals/8(res_vy_lowerlimit) -> Relational Operator7/2
  Logical Operator/1 -> Debounce1/1
  Logical Operator1/1 -> Debounce2/1
  Debounce2/1 -> Logical Operator2/2, SpeedResidualsOK/1
  Debounce1/1 -> Logical Operator2/1
  Logical Operator2/1 -> ResidualsOK/1

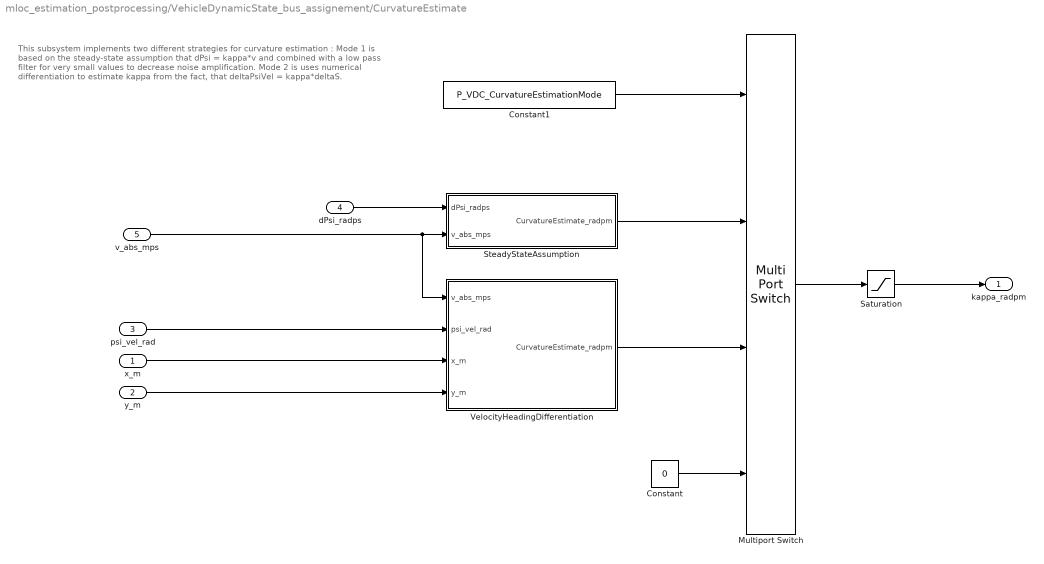
== system mloc_estimation_postprocessing/VehicleDynamicState_bus_assignement/CurvatureEstimate ==
  note: This subsystem implements two different strategies for curvature estimation :
      |
      | Mode 1 is based on the steady-state assumption that dPsi = kappa*v and combined
      | with a low pass filter for very small values to decrease noise amplification.
      |
      | Mode 2 is uses numerical differentiation to estimate kappa from the fact, that
      | deltaPsiVel = kappa*deltaS.
  "x_m " : Inport
  y_m : Inport  Port=2
  psi_vel_rad : Inport  Port=3
  dPsi_radps : Inport  Port=4
  v_abs_mps : Inport  Port=5
  Constant : Constant  Value=0
  Constant1 : Constant  Value=P_VDC_CurvatureEstimationMode
  Multiport Switch : MultiPortSwitch  Inputs=2  DataPortForDefault=Additional data port
  Saturation : Saturate  UpperLimit=P_VDC_CurvatureEstimateMax_radpm  LowerLimit=-P_VDC_CurvatureEstimateMax_radpm
  SteadyStateAssumption : Subsystem
  VelocityHeadingDifferentiation : Subsystem
  kappa_radpm : Outport
  wires:
  Constant/1 -> Multiport Switch/4
  dPsi_radps/1 -> SteadyStateAssumption/1(dPsi_radps)
  SteadyStateAssumption/1(CurvatureEstimate_radpm) -> Multiport Switch/2
  v_abs_mps/1 -> VelocityHeadingDifferentiation/1(v_abs_mps), SteadyStateAssumption/2(v_abs_mps)
  psi_vel_rad/1 -> VelocityHeadingDifferentiation/2(psi_vel_rad)
  "x_m "/1 -> VelocityHeadingDifferentiation/3("x_m ")
  y_m/1 -> VelocityHeadingDifferentiation/4(y_m)
  VelocityHeadingDifferentiation/1(CurvatureEstimate_radpm) -> Multiport Switch/3
  Constant1/1 -> Multiport Switch/1
  Multiport Switch/1 -> Saturation/1
  Saturation/1 -> kappa_radpm/1

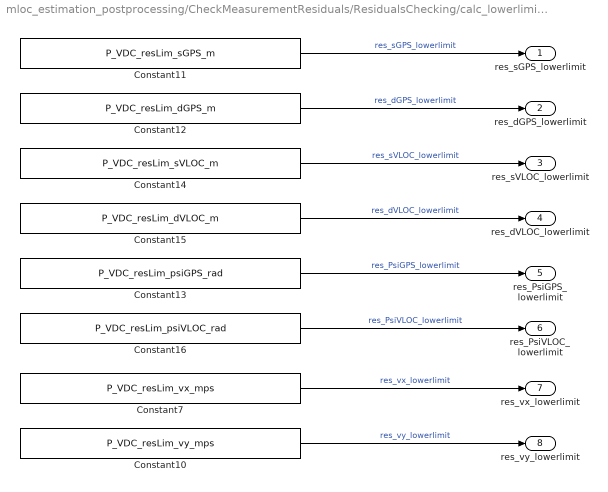
== system mloc_estimation_postprocessing/CheckMeasurementResiduals/ResidualsChecking/calc_lowerlimit_residuals ==
  Constant10 : Constant  Value=P_VDC_resLim_vy_mps
  Constant11 : Constant  Value=P_VDC_resLim_sGPS_m
  Constant12 : Constant  Value=P_VDC_resLim_dGPS_m
  Constant13 : Constant  Value=P_VDC_resLim_psiGPS_rad
  Constant14 : Constant  Value=P_VDC_resLim_sVLOC_m
  Constant15 : Constant  Value=P_VDC_resLim_dVLOC_m
  Constant16 : Constant  Value=P_VDC_resLim_psiVLOC_rad
  Constant7 : Constant  Value=P_VDC_resLim_vx_mps
  res_sGPS_lowerlimit : Outport
  res_dGPS_lowerlimit : Outport  Port=2
  res_sVLOC_lowerlimit : Outport  Port=3
  res_dVLOC_lowerlimit : Outport  Port=4
  res_PsiGPS_lowerlimit : Outport  Port=5
  res_PsiVLOC_lowerlimit : Outport  Port=6
  res_vx_lowerlimit : Outport  Port=7
  res_vy_lowerlimit : Outport  Port=8
  wires:
  Constant10/1 -> res_vy_lowerlimit/1  "res_vy_lowerlimit"
  Constant11/1 -> res_sGPS_lowerlimit/1  "res_sGPS_lowerlimit"
  Constant16/1 -> res_PsiVLOC_lowerlimit/1  "res_PsiVLOC_lowerlimit"
  Constant12/1 -> res_dGPS_lowerlimit/1  "res_dGPS_lowerlimit"
  Constant15/1 -> res_dVLOC_lowerlimit/1  "res_dVLOC_lowerlimit"
  Constant13/1 -> res_PsiGPS_lowerlimit/1  "res_PsiGPS_lowerlimit"
  Constant14/1 -> res_sVLOC_lowerlimit/1  "res_sVLOC_lowerlimit"
  Constant7/1 -> res_vx_lowerlimit/1  "res_vx_lowerlimit"

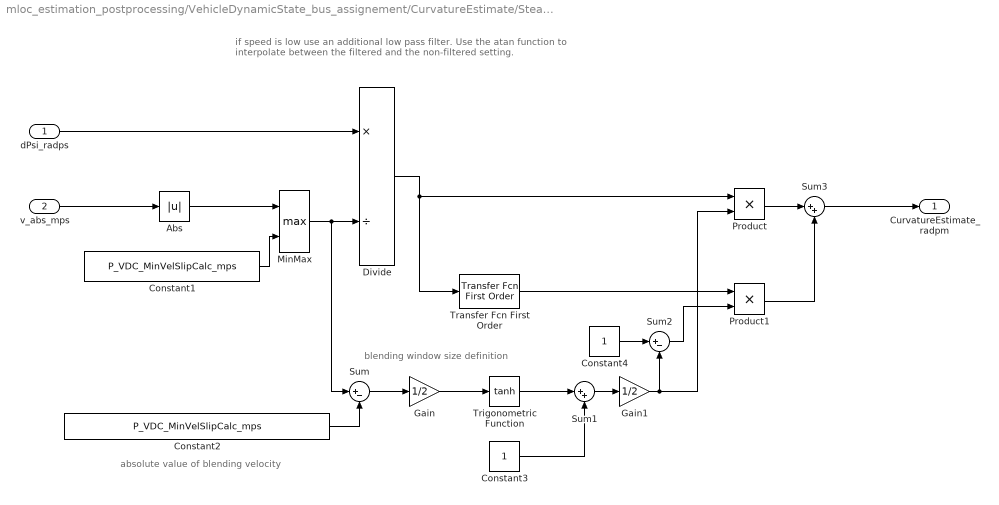
== system mloc_estimation_postprocessing/VehicleDynamicState_bus_assignement/CurvatureEstimate/SteadyStateAssumption ==
  note: blending window size definition
  note: absolute value of blending velocity
  note: if speed is low use an additional low pass filter.
      | Use the atan function to interpolate between the filtered and the non-filtered setting.
  dPsi_radps : Inport
  v_abs_mps : Inport  Port=2
  Abs : Abs
  Constant1 : Constant  Value=P_VDC_MinVelSlipCalc_mps
  Constant2 : Constant  Value=P_VDC_MinVelSlipCalc_mps
  Constant3 : Constant
  Constant4 : Constant
  Divide : Product  Inputs=*/
  Gain : Gain  Gain=1/2
  Gain1 : Gain  Gain=1/2
  MinMax : MinMax  Function=max  Inputs=2
  Product : Product
  Product1 : Product
  Sum : Sum  Inputs=|+-
  Sum1 : Sum  Inputs=|++
  Sum2 : Sum  Inputs=|+-
  Sum3 : Sum  Inputs=|++
  Transfer Fcn First Order : simulink/Discrete/Transfer Fcn First Order  PoleZ=exp(-tS/P_VDC_LowPassT1Curvature)  ICPrevOutput=0.0  DoSatur=off
      settings: SourceProductName=Simulink
  Trigonometric Function : Trigonometry  Operator=tanh
  CurvatureEstimate_radpm : Outport
  wires:
  Sum/1 -> Gain/1
  MinMax/1 -> Sum/1, Divide/2
  Constant1/1 -> MinMax/2
  Constant3/1 -> Sum1/2
  Divide/1 -> Transfer Fcn First Order/1, Product/1
  Constant4/1 -> Sum2/1
  Trigonometric Function/1 -> Sum1/1
  Gain/1 -> Trigonometric Function/1
  Constant2/1 -> Sum/2
  Abs/1 -> MinMax/1
  Product1/1 -> Sum3/2
  Sum1/1 -> Gain1/1
  Gain1/1 -> Product/2, Sum2/2
  Product/1 -> Sum3/1
  Sum2/1 -> Product1/2
  Transfer Fcn First Order/1 -> Product1/1
  v_abs_mps/1 -> Abs/1
  dPsi_radps/1 -> Divide/1
  Sum3/1 -> CurvatureEstimate_radpm/1

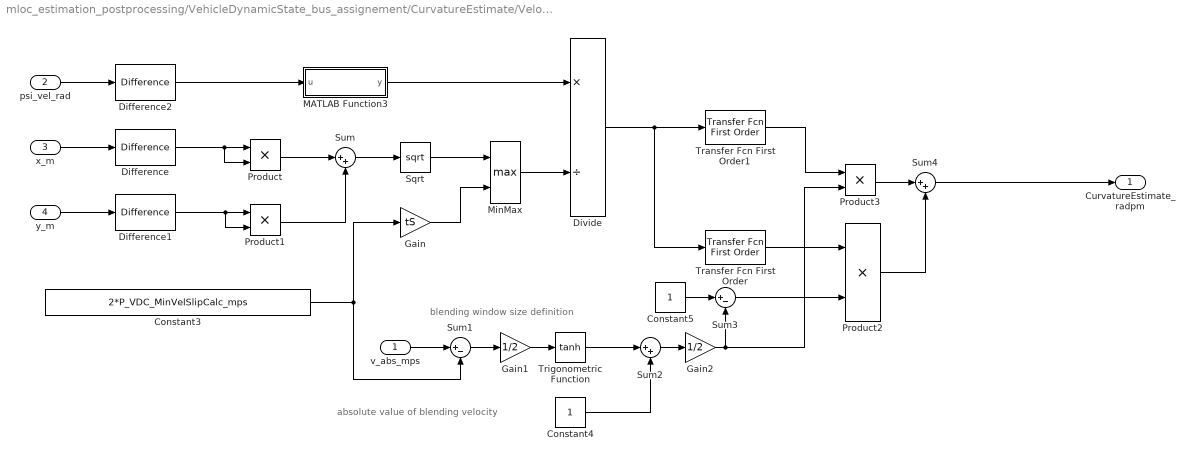
== system mloc_estimation_postprocessing/VehicleDynamicState_bus_assignement/CurvatureEstimate/VelocityHeadingDifferentiation ==
  note: absolute value of blending velocity
  note: blending window size definition
  v_abs_mps : Inport
  psi_vel_rad : Inport  Port=2
  "x_m " : Inport  Port=3
  y_m : Inport  Port=4
  Constant3 : Constant  Value=2*P_VDC_MinVelSlipCalc_mps
  Constant4 : Constant
  Constant5 : Constant
  Difference : simulink/Discrete/Difference  ICPrevInput=0.0  OutMin=[]  OutMax=[]  OutDataType=fixdt(1, 16)  OutScaling=2^-10  DoSatur=off
  Difference1 : simulink/Discrete/Difference  ICPrevInput=0.0  OutMin=[]  OutMax=[]  OutDataType=fixdt(1, 16)  OutScaling=2^-10  DoSatur=off
  Difference2 : simulink/Discrete/Difference  ICPrevInput=0.0  OutMin=[]  OutMax=[]  OutDataType=fixdt(1, 16)  OutScaling=2^-10  DoSatur=off
  Divide : Product  Inputs=*/
  Gain : Gain  Gain=tS
  Gain1 : Gain  Gain=1/2
  Gain2 : Gain  Gain=1/2
  MATLAB Function3 : MATLAB Function  TreatAsAtomicUnit=on
  MinMax : MinMax  Function=max  Inputs=2
  Product{,1..3} (4 alike) : Product
  Sqrt : Sqrt  SaturateOnIntegerOverflow=on
  Sum : Sum  Inputs=|++
  Sum1 : Sum  Inputs=|+-
  Sum2 : Sum  Inputs=|++
  Sum3 : Sum  Inputs=|+-
  Sum4 : Sum  Inputs=|++
  Transfer Fcn First Order : simulink/Discrete/Transfer Fcn First Order  PoleZ=exp(-tS/P_VDC_LowPassT1Curvature)  ICPrevOutput=0.0  DoSatur=off
      settings: SourceProductName=Simulink
  Transfer Fcn First Order1 : simulink/Discrete/Transfer Fcn First Order  PoleZ=exp(-tS/(0.5*P_VDC_LowPassT1Curvature))  ICPrevOutput=0.0  DoSatur=off
      settings: SourceProductName=Simulink
  Trigonometric Function : Trigonometry  Operator=tanh
  CurvatureEstimate_radpm : Outport
  wires:
  Difference1/1 -> Product1/2, Product1/1
  Difference/1 -> Product/2, Product/1
  Product1/1 -> Sum/2
  Transfer Fcn First Order/1 -> Product2/1
  Product/1 -> Sum/1
  MinMax/1 -> Divide/2
  Constant4/1 -> Sum2/2
  Difference2/1 -> MATLAB Function3/1(u)
  Sum2/1 -> Gain2/1
  Gain/1 -> MinMax/2
  Sum/1 -> Sqrt/1
  Constant3/1 -> Sum1/2, Gain/1
  Product2/1 -> Sum4/2
  y_m/1 -> Difference1/1
  "x_m "/1 -> Difference/1
  Sum3/1 -> Product2/2
  Gain1/1 -> Trigonometric Function/1
  Gain2/1 -> Product3/2, Sum3/2
  Constant5/1 -> Sum3/1
  v_abs_mps/1 -> Sum1/1
  psi_vel_rad/1 -> Difference2/1
  Trigonometric Function/1 -> Sum2/1
  Sum1/1 -> Gain1/1
  Sqrt/1 -> MinMax/1
  Product3/1 -> Sum4/1
  Divide/1 -> Transfer Fcn First Order/1, Transfer Fcn First Order1/1
  Sum4/1 -> CurvatureEstimate_radpm/1
  MATLAB Function3/1(y) -> Divide/1
  Transfer Fcn First Order1/1 -> Product3/1

== matlab function mloc_estimation_postprocessing/VehicleDynamicState_bus_assignement/MATLAB Function ==
  data: omega_rad input size=4; vxCB_mps input; vyCG_mps input; dPsi_radps input; DeltaWheel_rad input; lambda_perc output; alpha_rad output; tyreradius_rear_m parameter; tyreradius_front_m parameter; tw_rear_m parameter; tw_front_m parameter; l_rear_m parameter; l_front_m parameter; P_VDC_MinVelSlipCalc_mps parameter
function [lambda_perc, alpha_rad] = fcn(omega_rad, vxCB_mps, vyCG_mps, dPsi_radps, DeltaWheel_rad, tyreradius_rear_m, tyreradius_front_m, tw_rear_m, tw_front_m, l_rear_m, l_front_m, P_VDC_MinVelSlipCalc_mps)
%#codegen
  [lambda_perc, alpha_rad] = calcWheelSlips(omega_rad, [vxCB_mps; vyCG_mps; dPsi_radps], DeltaWheel_rad, tw_front_m, tw_rear_m, l_front_m, l_rear_m, tyreradius_front_m, tyreradius_rear_m, P_VDC_MinVelSlipCalc_mps);

== matlab function mloc_estimation_postprocessing/CalculateOdometry/IntegrateOdometry/MATLAB Function ==
  data: vx_mps input; Position output Bus: CartPos; vy_mps input; dPsi_rad input; OdometryPosition_old input Bus: CartPos; tS parameter
function Position  = fcn_integrateOdometry(vx_mps, vy_mps, dPsi_rad, OdometryPosition_old, tS)

[Position] = integrateOdometry(vx_mps, vy_mps, dPsi_rad, OdometryPosition_old, tS);

== matlab function mloc_estimation_postprocessing/VehicleDynamicState_bus_assignement/CurvatureEstimate/VelocityHeadingDifferentiation/MATLAB Function3 ==
  data: u input; y output
function y = fcn(u)

y = normalizeAngle(u);

== matlab function mloc_estimation_postprocessing/VehicleDynamicState_bus_assignement/MATLAB Function2 ==
  data: vx_mps input; dBeta_radps output; vy_mps input; ax_mps2 input; ay_mps2 input; dPsi_radps input
function dBeta_radps = fcn(vx_mps, vy_mps, ax_mps2, ay_mps2, dPsi_radps )
%#codegen

[ dBeta_radps ] = calc_dBeta( vx_mps, vy_mps, ax_mps2, ay_mps2, dPsi_radps );

== matlab function mloc_estimation_postprocessing/VehicleDynamicState_bus_assignement/MATLAB Function3 ==
  data: u input; y output
function y = fcn(u)

y = normalizeAngle(u);
